simulink library "lib_fuel_cell"  (Simulink 4.00)
undefined symbols (not defined in the file or in its folder): air_cp, amb_tmp, cell_const_F, cell_const_g, cell_const_jo, cell_const_LHV_H2, cell_const_Mair, cell_const_MH, cell_const_MW, cell_const_R2, cell_const_Voc, ex_gas_cp, fan_cool, fc_acc_mass, fc_act, fc_air_comp_map, fc_air_comp_pwr, fc_base_mass, fc_blower_rec_H2, fc_blowera, fc_c2i_th_cond, fc_c_init_tmp, fc_cell_area, fc_cell_const_eta1, fc_cell_const_eta_DCDC, fc_cell_const_etablow, fc_cell_const_etagen, fc_cell_const_etapump, fc_cell_const_ex, fc_cell_const_kw, fc_cell_const_Nrad, fc_cell_const_U, fc_cell_dim_A, fc_cell_dim_tm, fc_cell_num, fc_cell_press_a, fc_cell_press_amb, fc_cell_press_an, fc_cell_press_blowa, fc_cell_press_blowr, fc_cell_press_c, fc_cell_press_hum, fc_cell_press_hyd, fc_cell_stack_dpipe, fc_cell_stack_dpipefc, fc_cell_stack_drad, fc_cell_stack_Lpipe, fc_cell_stack_Lpipefc, fc_cell_stack_Lrad, fc_cell_stack_N, fc_cell_stack_Pel, fc_cell_stoich_RHah, fc_cell_stoich_RHch, fc_cell_stoich_RHo, fc_cell_stoich_vH, fc_cell_stoich_vO, fc_cell_stoich_XON, fc_cell_temp_ah, fc_cell_temp_amb, fc_cell_temp_cell ... (+74)
libraries: fc_vt_lib x2, lib_fuel_cell x1
(part 3 of 5)

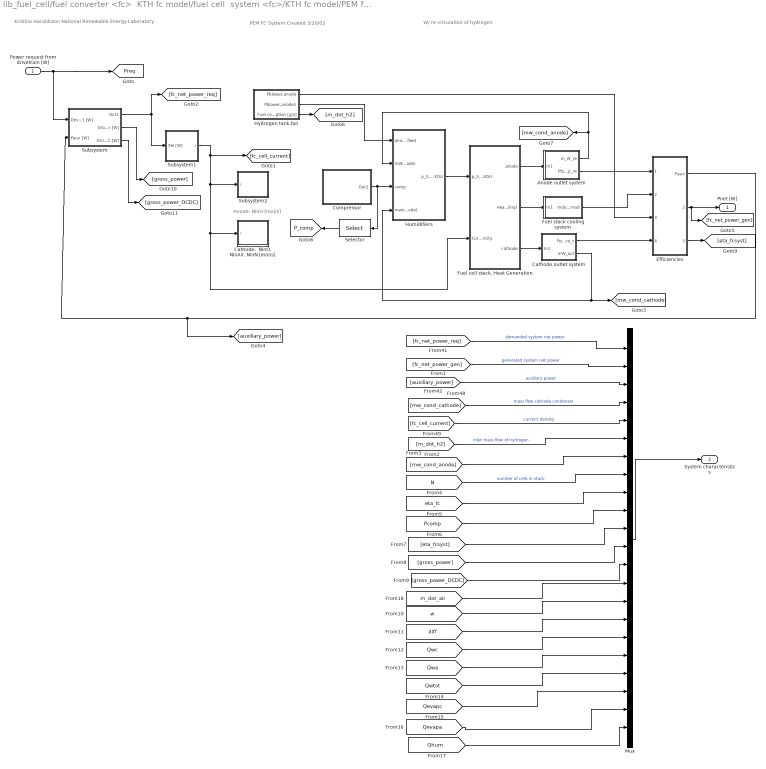
== system lib_fuel_cell/fuel converter <fc>  KTH fc model/fuel cell  system <fc>/KTH fc model/PEM fuel cell system ==
  note: Kristina Haraldsson
      | National Renewable Energy Laboratory
  note: PEM FC System
      | Created  3/20/02
  note: W/ re-circulation of hydrogen
  note: Anode: NinH [mol/s]
  "Power request from drivetrain [W] " : Inport  Port=1  LatchInput=off
  Anode outlet system : Subsystem
      settings: RTWFcnNameOpts=Auto  RTWFileNameOpts=Auto
  Cathode outlet system : Subsystem
      settings: RTWFcnNameOpts=Auto  RTWFileNameOpts=Auto
  "Cathode:  NinO, NinAir, NinN [mol/s]" : Subsystem
      settings: RTWFcnNameOpts=Auto  RTWFileNameOpts=Auto
  "Compressor " : Subsystem
      settings: RTWFcnNameOpts=Auto  RTWFileNameOpts=Auto
  Efficiencies : Subsystem
      settings: RTWFcnNameOpts=Auto  RTWFileNameOpts=Auto
  "Fuel cell stack, Heat Generation" : Subsystem
      settings: RTWFcnNameOpts=Auto  RTWFileNameOpts=Auto
  Fuel stack cooling system : Subsystem
      settings: RTWFcnNameOpts=Auto  RTWFileNameOpts=Auto
  Humidifiers : Subsystem
      settings: RTWFcnNameOpts=Auto  RTWFileNameOpts=Auto
  Hydrogen tank,fan : Subsystem
      settings: RTWFcnNameOpts=Auto  RTWFileNameOpts=Auto
  Mux : Mux  Inputs=22
  Selector : Selector  Orientation=left  InputType=Vector  ElementSrc=Internal  Elements=[4]  RowSrc=Internal  Rows=1  ColumnSrc=Internal  Columns=1  InputPortWidth=7
  Subsystem : Subsystem
      settings: RTWFcnNameOpts=Auto  RTWFileNameOpts=Auto
  Subsystem1 : Subsystem
      settings: RTWFcnNameOpts=Auto  RTWFileNameOpts=Auto
  Subsystem2 : Subsystem
      settings: RTWFcnNameOpts=Auto  RTWFileNameOpts=Auto
  Pnet [W] : Outport  Port=1
  System characteristics : Outport  Port=2
  tag scope: P_comp=global, Preq=global
  wires:
  Humidifiers/1("p_56 anode feed p_57 cathode feed Psat Psatah Psatch XWaI,  XWcI  XOcI ") -> "Fuel cell stack, Heat Generation"/1("p_56, NinH, p_57, NinAir, Psat,Psatah,PsatchXWaI, XWcI, XOcI")
  "Compressor "/1(Out2) -> Humidifiers/3(comp), Selector/1
  "Fuel cell stack, Heat Generation"/1(anode) -> Anode outlet system/1(In1)
  "Fuel cell stack, Heat Generation"/2(Heat_fc (fuel cell stack cooling)) -> Fuel stack cooling system/1(In1)
  Fuel stack cooling system/1(mdotW P_pump A Heat Qcool P_fanrad) -> Efficiencies/2(P_pump,cool P_fanrad)
  Anode outlet system/2(Pfan Ppump_re) -> Efficiencies/1("P_fan_,re, P_pump_re_a")
  Anode outlet system/1(m_W_re) -> Humidifiers/2(mW_out(anode)), [mw_cond_anode]
  "Fuel cell stack, Heat Generation"/3(cathode) -> Cathode outlet system/1(In1)
  Cathode outlet system/1(Ppump_re_c) -> Efficiencies/4(P_pump_re_c)
  Cathode outlet system/2(mW_out) -> Humidifiers/4(mwout(cathode)), [mw_cond_cathode]
  Hydrogen tank,fan/1(Pblower,anode) -> Efficiencies/3(P_fan,anode)
  Efficiencies/1(Paux) -> Subsystem/2(Paux [W]), [auxiliary_power]
  Subsystem/1(Out1) -> Subsystem1/1(Pel [W]), [fc_net_power_req]
  "Power request from drivetrain [W] "/1 -> Subsystem/1(Drivetrain Power Request [W]), [Preq]
  Subsystem1/1(i) -> Subsystem2/1(i), "Cathode:  NinO, NinAir, NinN [mol/s]"/1(i), "Fuel cell stack, Heat Generation"/2(Current density), [fc_cell_current]
  Hydrogen tank,fan/3(Fuel consumption [g/s]) -> [m_dot_h2]
  Hydrogen tank,fan/2(Pblower,anode1) -> Humidifiers/1(anode feed)
  [fc_net_power_req] -> Mux/1  "demanded system net power"
  [auxiliary_power] -> Mux/3  "auxiliary power"
  [mw_cond_cathode] -> Mux/4  "mass flow cathode condenser"
  [fc_cell_current] -> Mux/5  "current density"
  [fc_net_power_gen] -> Mux/2  "generated system net power"
  Mux/1 -> System characteristics/1
  [m_dot_h2] -> Mux/6  "inlet mass flow of hydrogen"
  [mw_cond_anode] -> Mux/7
  [N] -> Mux/8  "number of cells in stack"
  [eta_fc] -> Mux/9
  [Pcomp] -> Mux/10
  Selector/1 -> [P_comp]
  Subsystem/2(Gross power [W]) -> [gross_power]
  Efficiencies/2(Pnet [W]) -> Pnet [W]/1, [fc_net_power_gen]
  Efficiencies/3(eta_fcsyst) -> [eta_fcsyst]
  Subsystem/3(Gross power incl. DCDC [W]) -> [gross_power_DCDC]
  [eta_fcsyst] -> Mux/11
  [gross_power] -> Mux/12
  [gross_power_DCDC] -> Mux/13
  [Qhum] -> Mux/22
  [Qevapa] -> Mux/21
  [Qevapc] -> Mux/20
  [Qwtot] -> Mux/19
  [Qwa] -> Mux/18
  [Qwc] -> Mux/17
  [diff] -> Mux/16
  [w] -> Mux/15
  [m_dot_air] -> Mux/14

== system lib_fuel_cell/fuel converter <fc>  KTH fc model/fuel cell  system <fc>/KTH fc model/emissions info ==
  Block NOTES1 : Subsystem
      settings: RTWFcnNameOpts=Auto  RTWFileNameOpts=Auto
      mask Display: disp('Block\nNOTES')
  "CO, g/s1" : Ground
  Exhaust temp.=Cell temp. [C] : Constant  Value=fc_cell_temp_cell
  "HC, g/s2" : Ground
  Molecular weight H2 : Constant  Value=cell_const_MH
  Mux : Mux  Inputs=4
  Mux5 : Mux  Inputs=4
      settings: DisplayOption=none
  "NOx, g/s3" : Ground
  "O2, g/s" : Ground
  "PM, g/s4" : Ground
  Product : Product  Inputs=2  Multiplication=Element-wise(.*)  SaturateOnIntegerOverflow=on
  Sum : Sum  Inputs=|++  SaturateOnIntegerOverflow=on
  emission info CO HC NOx PM mass flow exhaust exhaust temperature O2 : Outport  Port=1  OutputWhenDisabled=reset  InitialOutput=eps
  wires:
  "O2, g/s"/1 -> Mux5/4
  Exhaust temp.=Cell temp. [C]/1 -> Mux5/3
  Mux5/1 -> emission info CO HC NOx PM mass flow exhaust exhaust temperature O2/1
  "CO, g/s1"/1 -> Mux/1
  Mux/1 -> Mux5/1
  "HC, g/s2"/1 -> Mux/2
  "NOx, g/s3"/1 -> Mux/3
  "PM, g/s4"/1 -> Mux/4
  Molecular weight H2/1 -> Product/1
  [Exhaust_a_hydrogen] -> Product/2
  Product/1 -> Sum/1
  [Exhaust_a_water] -> Sum/2
  Sum/1 -> Mux5/2

== system lib_fuel_cell/fuel converter <fc> GCTool linkage/fuel cell  system <fc>/GCTool fuel cell model/GCTool  Fuel Cell Model ==
  In1 : Inport  Port=1  LatchInput=off
  S-Function : S-Function  FunctionName=sfun_gctool_fuelcell  PortCounts=[]  SFunctionModules=''
  Out1 : Outport  Port=1  InitialOutput=0
  wires:
  S-Function/1 -> Out1/1
  In1/1 -> S-Function/1

== system lib_fuel_cell/fuel converter <fc> GCTool linkage/fuel use and EO emis Fuel Cell/fc temp/Block NOTES ==
  note: This block models the thermal behavior internal combustion engine (ICE).
      | Emphasis is on the coolant since this temperature is used to correct engine
      | fuel use.

== system lib_fuel_cell/fuel converter <fc> GCTool linkage/fuel use and EO emis Fuel Cell/fc temp/fc coolant ==
  Tcl : Inport  Port=1  LatchInput=off
  "Qfc_i " : Inport  Port=2  LatchInput=off
  Enable : EnablePort  StatesWhenEnabling=reset
  Constant : Constant  Value=fc_tstat
  Product1 : Product  Inputs=2  Multiplication=Element-wise(.*)  SaturateOnIntegerOverflow=on
  Qhtr : Fcn  Expr=fc_cl2h_eff*fc_h_air_flow*air_cp*(u - amb_tmp)
  Qi : Sum  Inputs=-+  SaturateOnIntegerOverflow=on
  Relational Operator : RelationalOperator  Operator=<=
  Qfc_rad : Outport  Port=1  OutputWhenDisabled=reset  InitialOutput=0
  Qfc_htr : Outport  Port=2  OutputWhenDisabled=reset  InitialOutput=0
  wires:
  Tcl/1 -> Qhtr/1, Relational Operator/2
  Relational Operator/1 -> Product1/1
  Constant/1 -> Relational Operator/1
  Product1/1 -> Qfc_rad/1
  "Qfc_i "/1 -> Qi/2
  Qhtr/1 -> Qi/1, Qfc_htr/1
  Qi/1 -> Product1/2

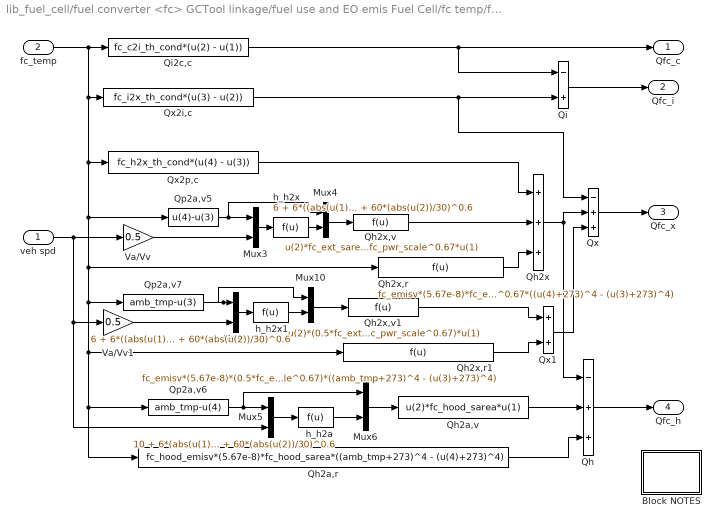
== system lib_fuel_cell/fuel converter <fc> GCTool linkage/fuel use and EO emis Fuel Cell/fc temp/fc mass heat flow ==
  veh spd : Inport  Port=1  LatchInput=off
  fc_temp : Inport  Port=2  LatchInput=off
  Block NOTES : Subsystem
      settings: RTWFcnNameOpts=Auto  RTWFileNameOpts=Auto
      mask Display: disp('Block\nNOTES')
  Mux{3..6,9..10} (6 alike) : Mux  Inputs=2
      settings: DisplayOption=none
  Qh : Sum  Inputs=-++  SaturateOnIntegerOverflow=on
  Qh2a,r : Fcn  Expr=fc_hood_emisv*(5.67e-8)*fc_hood_sarea*((amb_tmp+273)^4 - (u(4)+273)^4)
  Qh2a,v : Fcn  Expr=u(2)*fc_hood_sarea*u(1)
  Qh2x : Sum  Inputs=+++  SaturateOnIntegerOverflow=on
  Qh2x,r : Fcn  Expr=fc_emisv*(5.67e-8)*fc_ext_sarea*fc_pwr_scale^0.67*((u(4)+273)^4 - (u(3)+273)^4)
  Qh2x,r1 : Fcn  Expr=fc_emisv*(5.67e-8)*(0.5*fc_ext_sarea*fc_pwr_scale^0.67)*((amb_tmp+273)^4 - (u(3)+273)^4)
  Qh2x,v : Fcn  Expr=u(2)*fc_ext_sarea*fc_pwr_scale^0.67*u(1)
  Qh2x,v1 : Fcn  Expr=u(2)*(0.5*fc_ext_sarea*fc_pwr_scale^0.67)*u(1)
  Qi : Sum  Inputs=-+  SaturateOnIntegerOverflow=on
  Qi2c,c : Fcn  Expr=fc_c2i_th_cond*(u(2) - u(1))
  Qp2a,v5 : Fcn  Expr=u(4)-u(3)
  Qp2a,v6 : Fcn  Expr=amb_tmp-u(4)
  Qp2a,v7 : Fcn  Expr=amb_tmp-u(3)
  Qx : Sum  Inputs=-++  SaturateOnIntegerOverflow=on
  Qx1 : Sum  Inputs=++  SaturateOnIntegerOverflow=on
  Qx2i,c : Fcn  Expr=fc_i2x_th_cond*(u(3) - u(2))
  Qx2p,c : Fcn  Expr=fc_h2x_th_cond*(u(4) - u(3))
  Va/Vv : Gain  Gain=0.5  Multiplication=Element-wise(K.*u)  SaturateOnIntegerOverflow=on
  Va/Vv1 : Gain  Gain=0.5  Multiplication=Element-wise(K.*u)  SaturateOnIntegerOverflow=on
  h_h2a : Fcn  Expr=10 + 6*(abs(u(1))/1000)^0.3 + 60*(abs(u(2))/30)^0.6
  h_h2x : Fcn  Expr=6 + 6*((abs(u(1))/1000))^0.3 + 60*(abs(u(2))/30)^0.6
  h_h2x1 : Fcn  Expr=6 + 6*((abs(u(1))/1000))^0.3 + 60*(abs(u(2))/30)^0.6
  Qfc_c : Outport  Port=1
  Qfc_i : Outport  Port=2
  Qfc_x : Outport  Port=3
  Qfc_h : Outport  Port=4
  wires:
  Mux10/1 -> Qh2x,v1/1
  Mux9/1 -> h_h2x1/1
  Qp2a,v7/1 -> Mux9/1, Mux10/1
  h_h2x1/1 -> Mux10/2
  Va/Vv1/1 -> Mux9/2
  Mux4/1 -> Qh2x,v/1
  Mux3/1 -> h_h2x/1
  Qp2a,v5/1 -> Mux3/1, Mux4/1
  h_h2x/1 -> Mux4/2
  veh spd/1 -> Va/Vv/1, Mux5/2, Va/Vv1/1
  Va/Vv/1 -> Mux3/2
  Qi2c,c/1 -> Qfc_c/1, Qi/1
  fc_temp/1 -> Qx2p,c/1, Qh2x,r/1, Qp2a,v7/1, Qp2a,v6/1, Qh2a,r/1, Qh2x,r1/1, Qp2a,v5/1, Qx2i,c/1, Qi2c,c/1
  Qx2i,c/1 -> Qi/2, Qx/1
  Qi/1 -> Qfc_i/1
  Qx/1 -> Qfc_x/1
  Qh2x/1 -> Qx/2, Qh/1
  Qh/1 -> Qfc_h/1
  Mux6/1 -> Qh2a,v/1
  Mux5/1 -> h_h2a/1
  Qp2a,v6/1 -> Mux5/1, Mux6/1
  h_h2a/1 -> Mux6/2
  Qx1/1 -> Qx/3
  Qh2x,v/1 -> Qh2x/2
  Qx2p,c/1 -> Qh2x/1
  Qh2x,r1/1 -> Qx1/2
  Qh2x,v1/1 -> Qx1/1
  Qh2a,r/1 -> Qh/3
  Qh2a,v/1 -> Qh/2
  Qh2x,r/1 -> Qh2x/3

== system lib_fuel_cell/fuel converter <fc> GCTool linkage/fuel use and EO emis Fuel Cell/fc temp/old fc coolant  temp. (C) ==
  fc on? : Inport  Port=1  LatchInput=off
  veh spd : Inport  Port=2  LatchInput=off
  Block NOTES : Subsystem
      settings: RTWFcnNameOpts=Auto  RTWFileNameOpts=Auto
      mask Display: disp('Block\nNOTES')
  Mux : Mux  Inputs=4
      settings: DisplayOption=none
  TEC : Integrator  ExternalReset=none  InitialConditionSource=internal  InitialCondition=fc_i_init_tmp  LimitOutput=off  UpperSaturationLimit=inf  LowerSaturationLimit=-inf  ShowSaturationPort=off  ShowStatePort=off  AbsoluteTolerance=auto
  compute engine dT/dt : Fcn  Expr=1.1*u[1]*(-u[2]/218)*(95-u[4])+(1-u[1])*u[3]*(u[4]-amb_tmp)
  gamma (takes v as input) : Fcn  Expr=(-8.22e-5*u+8.09e-6*4-1.45e-4)*.45
  log(1-40/75) : Constant  Value=-0.7621
  fc coolant  temp (C) : Outport  Port=1  InitialOutput=0
  wires:
  compute engine dT/dt/1 -> TEC/1
  gamma (takes v as input)/1 -> Mux/3
  log(1-40/75)/1 -> Mux/2
  Mux/1 -> compute engine dT/dt/1
  fc on?/1 -> Mux/1
  veh spd/1 -> gamma (takes v as input)/1
  TEC/1 -> fc coolant  temp (C)/1, Mux/4

== system lib_fuel_cell/fuel converter <fc> VT model/Fuel Cell Power System Model (S. Gurski - Virgina Tech)/Fuel Cell System/Algebraic Constraint ==
  f(z) : Inport  Port=1  LatchInput=off
  Initial Guess : InitialCondition  Value=z0
  Sum : Sum  Inputs=|++  SaturateOnIntegerOverflow=on
  z : Outport  Port=1
  wires:
  Sum/1 -> Initial Guess/1
  Initial Guess/1 -> Sum/2, z/1
  f(z)/1 -> Sum/1

== system lib_fuel_cell/fuel converter <fc> VT model/Fuel Cell Power System Model (S. Gurski - Virgina Tech)/Fuel Cell System/Fuel Cell System ==
  " Current Density Request" : Inport  Port=1  LatchInput=off
  t_stack_coolant_in1 : Inport  Port=2  LatchInput=off
  fc_stack_temperature : Inport  Port=3  LatchInput=off
  water_balance_previous : Inport  Port=4  LatchInput=off
  elevation : Inport  Port=5  LatchInput=off
  vehicle speed (m/s) : Inport  Port=6  LatchInput=off
  Main Loop : fc_vt_lib/Main Loop
      settings: RTWFcnNameOpts=Auto  RTWFileNameOpts=Auto
  Net Power Gen : Outport  Port=1
  Stack Temperature : Outport  Port=2
  cell_voltage : Outport  Port=3
  t_stack_coolant_in : Outport  Port=4
  waterbalance : Outport  Port=5
  system_characteristics : Outport  Port=6
  wires:
  elevation/1 -> Main Loop/5
  Main Loop/6 -> system_characteristics/1
  water_balance_previous/1 -> Main Loop/4
  fc_stack_temperature/1 -> Main Loop/3
  t_stack_coolant_in1/1 -> Main Loop/2
  Main Loop/5 -> cell_voltage/1
  " Current Density Request"/1 -> Main Loop/1
  Main Loop/2 -> waterbalance/1
  Main Loop/3 -> Stack Temperature/1
  Main Loop/4 -> t_stack_coolant_in/1
  Main Loop/1 -> Net Power Gen/1
  vehicle speed (m/s)/1 -> Main Loop/6

== system lib_fuel_cell/fuel converter <fc> net model/fuel cell  system <fc>/pwr vs. eff  fuel cell model/enforce limits ==
  In1 : Inport  Port=1  LatchInput=off
  Saturation : Saturate  UpperLimit=max(fc_pwr_map)*fc_pwr_scale  LowerLimit=0  LinearizeAsGain=on
  Out1 : Outport  Port=1  InitialOutput=0
  wires:
  In1/1 -> Saturation/1
  Saturation/1 -> Out1/1

== system lib_fuel_cell/fuel converter <fc> net model/fuel use and EO emis Fuel Cell/HOT engine maps /Block NOTES ==
  note: This block determines the fully hot fuel use, engine-out emissions output rates, exhaust gas mass flow rate,
      | and engine-out exhaust gas temperature as a function of engine output torque and speed.
      | The engine maps (except for exhaust gas temperature) can be scaled using variables fc_spd_scale and
      |  fc_trq_scale; it is recommended that scaling values outside the range of 0.85 to 1.15 be used CAREFULLY.

== system lib_fuel_cell/fuel converter <fc> net model/fuel use and EO emis Fuel Cell/fc temp/Block NOTES ==
  note: This block models the thermal behavior internal combustion engine (ICE).
      | Emphasis is on the coolant since this temperature is used to correct engine
      | fuel use.

== system lib_fuel_cell/fuel converter <fc> net model/fuel use and EO emis Fuel Cell/fc temp/fc coolant ==
  Tcl : Inport  Port=1  LatchInput=off
  "Qfc_i " : Inport  Port=2  LatchInput=off
  Enable : EnablePort  StatesWhenEnabling=reset
  Constant : Constant  Value=fc_tstat
  Product1 : Product  Inputs=2  Multiplication=Element-wise(.*)  SaturateOnIntegerOverflow=on
  Qhtr : Fcn  Expr=fc_cl2h_eff*fc_h_air_flow*air_cp*(u - amb_tmp)
  Qi : Sum  Inputs=-+  SaturateOnIntegerOverflow=on
  Relational Operator : RelationalOperator  Operator=<=
  Qfc_rad : Outport  Port=1  OutputWhenDisabled=reset  InitialOutput=0
  Qfc_htr : Outport  Port=2  OutputWhenDisabled=reset  InitialOutput=0
  wires:
  Tcl/1 -> Qhtr/1, Relational Operator/2
  Relational Operator/1 -> Product1/1
  Constant/1 -> Relational Operator/1
  Product1/1 -> Qfc_rad/1
  "Qfc_i "/1 -> Qi/2
  Qhtr/1 -> Qi/1, Qfc_htr/1
  Qi/1 -> Product1/2

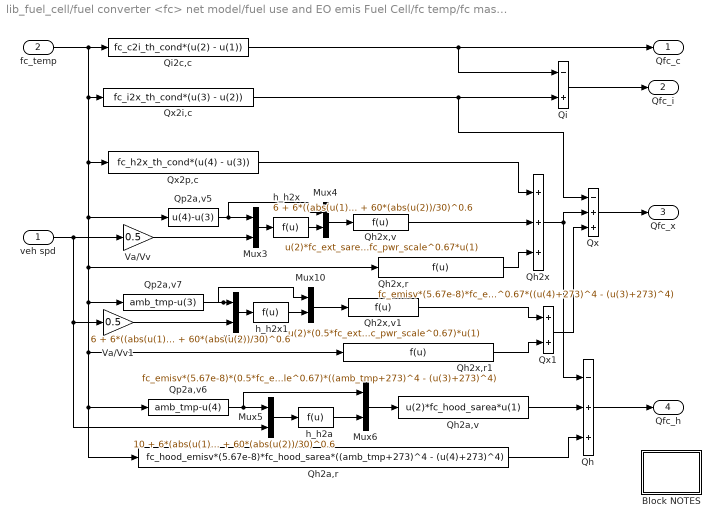
== system lib_fuel_cell/fuel converter <fc> net model/fuel use and EO emis Fuel Cell/fc temp/fc mass heat flow ==
  veh spd : Inport  Port=1  LatchInput=off
  fc_temp : Inport  Port=2  LatchInput=off
  Block NOTES : Subsystem
      settings: RTWFcnNameOpts=Auto  RTWFileNameOpts=Auto
      mask Display: disp('Block\nNOTES')
  Mux{3..6,9..10} (6 alike) : Mux  Inputs=2
      settings: DisplayOption=none
  Qh : Sum  Inputs=-++  SaturateOnIntegerOverflow=on
  Qh2a,r : Fcn  Expr=fc_hood_emisv*(5.67e-8)*fc_hood_sarea*((amb_tmp+273)^4 - (u(4)+273)^4)
  Qh2a,v : Fcn  Expr=u(2)*fc_hood_sarea*u(1)
  Qh2x : Sum  Inputs=+++  SaturateOnIntegerOverflow=on
  Qh2x,r : Fcn  Expr=fc_emisv*(5.67e-8)*fc_ext_sarea*fc_pwr_scale^0.67*((u(4)+273)^4 - (u(3)+273)^4)
  Qh2x,r1 : Fcn  Expr=fc_emisv*(5.67e-8)*(0.5*fc_ext_sarea*fc_pwr_scale^0.67)*((amb_tmp+273)^4 - (u(3)+273)^4)
  Qh2x,v : Fcn  Expr=u(2)*fc_ext_sarea*fc_pwr_scale^0.67*u(1)
  Qh2x,v1 : Fcn  Expr=u(2)*(0.5*fc_ext_sarea*fc_pwr_scale^0.67)*u(1)
  Qi : Sum  Inputs=-+  SaturateOnIntegerOverflow=on
  Qi2c,c : Fcn  Expr=fc_c2i_th_cond*(u(2) - u(1))
  Qp2a,v5 : Fcn  Expr=u(4)-u(3)
  Qp2a,v6 : Fcn  Expr=amb_tmp-u(4)
  Qp2a,v7 : Fcn  Expr=amb_tmp-u(3)
  Qx : Sum  Inputs=-++  SaturateOnIntegerOverflow=on
  Qx1 : Sum  Inputs=++  SaturateOnIntegerOverflow=on
  Qx2i,c : Fcn  Expr=fc_i2x_th_cond*(u(3) - u(2))
  Qx2p,c : Fcn  Expr=fc_h2x_th_cond*(u(4) - u(3))
  Va/Vv : Gain  Gain=0.5  Multiplication=Element-wise(K.*u)  SaturateOnIntegerOverflow=on
  Va/Vv1 : Gain  Gain=0.5  Multiplication=Element-wise(K.*u)  SaturateOnIntegerOverflow=on
  h_h2a : Fcn  Expr=10 + 6*(abs(u(1))/1000)^0.3 + 60*(abs(u(2))/30)^0.6
  h_h2x : Fcn  Expr=6 + 6*((abs(u(1))/1000))^0.3 + 60*(abs(u(2))/30)^0.6
  h_h2x1 : Fcn  Expr=6 + 6*((abs(u(1))/1000))^0.3 + 60*(abs(u(2))/30)^0.6
  Qfc_c : Outport  Port=1
  Qfc_i : Outport  Port=2
  Qfc_x : Outport  Port=3
  Qfc_h : Outport  Port=4
  wires:
  Mux10/1 -> Qh2x,v1/1
  Mux9/1 -> h_h2x1/1
  Qp2a,v7/1 -> Mux9/1, Mux10/1
  h_h2x1/1 -> Mux10/2
  Va/Vv1/1 -> Mux9/2
  Mux4/1 -> Qh2x,v/1
  Mux3/1 -> h_h2x/1
  Qp2a,v5/1 -> Mux3/1, Mux4/1
  h_h2x/1 -> Mux4/2
  veh spd/1 -> Va/Vv/1, Mux5/2, Va/Vv1/1
  Va/Vv/1 -> Mux3/2
  Qi2c,c/1 -> Qfc_c/1, Qi/1
  fc_temp/1 -> Qx2p,c/1, Qh2x,r/1, Qp2a,v7/1, Qp2a,v6/1, Qh2a,r/1, Qh2x,r1/1, Qp2a,v5/1, Qx2i,c/1, Qi2c,c/1
  Qx2i,c/1 -> Qi/2, Qx/1
  Qi/1 -> Qfc_i/1
  Qx/1 -> Qfc_x/1
  Qh2x/1 -> Qx/2, Qh/1
  Qh/1 -> Qfc_h/1
  Mux6/1 -> Qh2a,v/1
  Mux5/1 -> h_h2a/1
  Qp2a,v6/1 -> Mux5/1, Mux6/1
  h_h2a/1 -> Mux6/2
  Qx1/1 -> Qx/3
  Qh2x,v/1 -> Qh2x/2
  Qx2p,c/1 -> Qh2x/1
  Qh2x,r1/1 -> Qx1/2
  Qh2x,v1/1 -> Qx1/1
  Qh2a,r/1 -> Qh/3
  Qh2a,v/1 -> Qh/2
  Qh2x,r/1 -> Qh2x/3

== system lib_fuel_cell/fuel converter <fc> net model/fuel use and EO emis Fuel Cell/fc temp/old fc coolant  temp. (C) ==
  fc on? : Inport  Port=1  LatchInput=off
  veh spd : Inport  Port=2  LatchInput=off
  Block NOTES : Subsystem
      settings: RTWFcnNameOpts=Auto  RTWFileNameOpts=Auto
      mask Display: disp('Block\nNOTES')
  Mux : Mux  Inputs=4
      settings: DisplayOption=none
  TEC : Integrator  ExternalReset=none  InitialConditionSource=internal  InitialCondition=fc_i_init_tmp  LimitOutput=off  UpperSaturationLimit=inf  LowerSaturationLimit=-inf  ShowSaturationPort=off  ShowStatePort=off  AbsoluteTolerance=auto
  compute engine dT/dt : Fcn  Expr=1.1*u[1]*(-u[2]/218)*(95-u[4])+(1-u[1])*u[3]*(u[4]-amb_tmp)
  gamma (takes v as input) : Fcn  Expr=(-8.22e-5*u+8.09e-6*4-1.45e-4)*.45
  log(1-40/75) : Constant  Value=-0.7621
  fc coolant  temp (C) : Outport  Port=1  InitialOutput=0
  wires:
  compute engine dT/dt/1 -> TEC/1
  gamma (takes v as input)/1 -> Mux/3
  log(1-40/75)/1 -> Mux/2
  Mux/1 -> compute engine dT/dt/1
  fc on?/1 -> Mux/1
  veh spd/1 -> gamma (takes v as input)/1
  TEC/1 -> fc coolant  temp (C)/1, Mux/4

== system lib_fuel_cell/fuel converter <fc> net model/fuel use and EO emis Fuel Cell/fc temp correct/fc temp correct Constant Correction Factors (Equation Based) ==
  Coolant T (C) : Inport  Port=1  LatchInput=off
  HOT fuel use (g/s) : Inport  Port=2  LatchInput=off
  HOT emis (g/s) : Inport  Port=3  LatchInput=off
  Enable : EnablePort  StatesWhenEnabling=reset
  Block NOTES : Subsystem
      settings: RTWFcnNameOpts=Auto  RTWFileNameOpts=Auto
      mask Display: disp('Block\nNOTES')
  CO cold/hot : Fcn  Expr=2.13*pow(u,4.26)+1
  HC cold/hot : Fcn  Expr=8.05*pow(u,9.46)+1
  Mux : Mux  Inputs=4
      settings: DisplayOption=none
  NOx cold/hot : Fcn  Expr=0.51*pow(u,1.37)+1
  PM cold/hot : Fcn  Expr=5.14*pow(u,17.04)+1
  Product : Product  Inputs=2  Multiplication=Element-wise(.*)  SaturateOnIntegerOverflow=on
  Product1 : Product  Inputs=2  Multiplication=Element-wise(.*)  SaturateOnIntegerOverflow=on
  Saturation : Saturate  UpperLimit=1  LowerLimit=0  LinearizeAsGain=on
  fuel cold/hot : Fcn  Expr=0.1*pow(u,0.65)+1
  lambda : Fcn  Expr=(fc_tstat-u)/(fc_tstat-20)
  fuel use (g/s) : Outport  Port=1  OutputWhenDisabled=reset  InitialOutput=0
  EO emis (g/s) : Outport  Port=2  OutputWhenDisabled=reset  InitialOutput=0
  wires:
  HOT emis (g/s)/1 -> Product/2
  Coolant T (C)/1 -> lambda/1
  HOT fuel use (g/s)/1 -> Product1/1
  Product1/1 -> fuel use (g/s)/1
  CO cold/hot/1 -> Mux/2
  Product/1 -> EO emis (g/s)/1
  fuel cold/hot/1 -> Product1/2
  Mux/1 -> Product/1
  lambda/1 -> Saturation/1
  Saturation/1 -> PM cold/hot/1, NOx cold/hot/1, fuel cold/hot/1, HC cold/hot/1, CO cold/hot/1
  HC cold/hot/1 -> Mux/1
  NOx cold/hot/1 -> Mux/3
  PM cold/hot/1 -> Mux/4

== system lib_fuel_cell/fuel converter <fc> net model/fuel use and EO emis Fuel Cell/fc temp correct/fc temp correct Variable Correction Factors (Map Based) ==
  Coolant T (C) : Inport  Port=1  LatchInput=off
  HOT fuel use (g/s) : Inport  Port=2  LatchInput=off
  HOT emis (g/s) : Inport  Port=3  LatchInput=off
  P (W) : Inport  Port=4  LatchInput=off
  Enable : EnablePort  StatesWhenEnabling=reset
  (Thot-Temp) -------------------- (Thot-Tcold) : Fcn  Expr=(fc_tstat-u)/(fc_tstat-fc_cold_tmp)
  CO factor cold-to-hot : Lookup  InputValues=fc_pwr_map*fc_pwr_scale  OutputValues=fc_co_map_c2h
  HC factor cold-to-hot : Lookup  InputValues=fc_pwr_map*fc_pwr_scale  OutputValues=fc_hc_map_c2h
  Mux{1..5} (5 alike) : Mux  Inputs=2
      settings: DisplayOption=none
  Mux6 : Mux  Inputs=4
      settings: DisplayOption=none
  NOx factor cold-to-hot : Lookup  InputValues=fc_pwr_map*fc_pwr_scale  OutputValues=fc_nox_map_c2h
  PM factor cold-to-hot : Lookup  InputValues=fc_pwr_map*fc_pwr_scale  OutputValues=fc_pm_map_c2h
  Product : Product  Inputs=2  Multiplication=Element-wise(.*)  SaturateOnIntegerOverflow=on
  Product1 : Product  Inputs=2  Multiplication=Element-wise(.*)  SaturateOnIntegerOverflow=on
  Saturation : Saturate  UpperLimit=max(fc_pwr_map*fc_pwr_scale)  LowerLimit=0  LinearizeAsGain=on
  cold/hot =1+(factor-1) *Temp_ratio{,1..4} (5 alike) : Fcn  Expr=1+(u[2]-1)*u[1]
  fuel factor cold-to-hot : Lookup  InputValues=fc_pwr_map*fc_pwr_scale  OutputValues=fc_fuel_map_c2h
  limit to data limits : Saturate  UpperLimit=1  LowerLimit=0  LinearizeAsGain=on
  fuel use (g/s) : Outport  Port=1  OutputWhenDisabled=reset  InitialOutput=0
  EO emis (g/s) : Outport  Port=2  OutputWhenDisabled=reset  InitialOutput=0
  wires:
  cold/hot =1+(factor-1) *Temp_ratio4/1 -> Mux6/4
  cold/hot =1+(factor-1) *Temp_ratio3/1 -> Mux6/3
  cold/hot =1+(factor-1) *Temp_ratio2/1 -> Mux6/2
  cold/hot =1+(factor-1) *Temp_ratio1/1 -> Mux6/1
  cold/hot =1+(factor-1) *Temp_ratio/1 -> Product1/2
  limit to data limits/1 -> Mux1/1, Mux2/1, Mux3/1, Mux4/1, Mux5/1
  (Thot-Temp) -------------------- (Thot-Tcold)/1 -> limit to data limits/1
  Saturation/1 -> PM factor cold-to-hot/1, NOx factor cold-to-hot/1, CO factor cold-to-hot/1, HC factor cold-to-hot/1, fuel factor cold-to-hot/1
  P (W)/1 -> Saturation/1
  HOT fuel use (g/s)/1 -> Product1/1
  Coolant T (C)/1 -> (Thot-Temp) -------------------- (Thot-Tcold)/1
  fuel factor cold-to-hot/1 -> Mux1/2
  Mux1/1 -> cold/hot =1+(factor-1) *Temp_ratio/1
  HC factor cold-to-hot/1 -> Mux2/2
  CO factor cold-to-hot/1 -> Mux3/2
  NOx factor cold-to-hot/1 -> Mux4/2
  PM factor cold-to-hot/1 -> Mux5/2
  Mux2/1 -> cold/hot =1+(factor-1) *Temp_ratio1/1
  Mux3/1 -> cold/hot =1+(factor-1) *Temp_ratio2/1
  Mux4/1 -> cold/hot =1+(factor-1) *Temp_ratio3/1
  Mux5/1 -> cold/hot =1+(factor-1) *Temp_ratio4/1
  Product1/1 -> fuel use (g/s)/1
  Product/1 -> EO emis (g/s)/1
  HOT emis (g/s)/1 -> Product/2
  Mux6/1 -> Product/1

== system lib_fuel_cell/fuel converter <fc> polarization curve model/fuel cell  system <fc>/polarization curve fuel cell model/Auxilaries  (actual) ==
  In1 : Inport  Port=1  LatchInput=off
  Air Compressor : Subsystem
      settings: RTWFcnNameOpts=Auto  RTWFileNameOpts=Auto
  Coolant Pump : Subsystem
      settings: RTWFcnNameOpts=Auto  RTWFileNameOpts=Auto
  Fuel Pump : Subsystem
      settings: RTWFcnNameOpts=Auto  RTWFileNameOpts=Auto
  Mux : Mux  Inputs=4
  Water Pump : Subsystem
      settings: RTWFcnNameOpts=Auto  RTWFileNameOpts=Auto
  pwr sum1 : Sum  Inputs=++++  SaturateOnIntegerOverflow=on
  Out1 : Outport  Port=1  InitialOutput=0
  Out2 : Outport  Port=2  InitialOutput=0
  wires:
  Water Pump/1(water pump  pwr request (W)) -> pwr sum1/3, Mux/3
  Coolant Pump/1(coolant pump  pwr request (W)) -> pwr sum1/4, Mux/4
  Air Compressor/1(air compressor  pwr request (W)) -> pwr sum1/2, Mux/2
  Fuel Pump/1(fuel pump  pwr request (W)) -> pwr sum1/1, Mux/1
  pwr sum1/1 -> Out1/1
  In1/1 -> Air Compressor/1(Fuel req'd (g/s)), Fuel Pump/1(Fuel req'd (g/s)), Water Pump/1(Fuel req'd (g/s))
  Mux/1 -> Out2/1

== system lib_fuel_cell/fuel converter <fc> polarization curve model/fuel cell  system <fc>/polarization curve fuel cell model/Auxilaries  (estimated) ==
  prev fuel  req (g/s) : Inport  Port=1  LatchInput=off
  Air Compressor : Subsystem
      settings: RTWFcnNameOpts=Auto  RTWFileNameOpts=Auto
  Coolant Pump : Subsystem
      settings: RTWFcnNameOpts=Auto  RTWFileNameOpts=Auto
  Fuel Pump : Subsystem
      settings: RTWFcnNameOpts=Auto  RTWFileNameOpts=Auto
  Water Pump : Subsystem
      settings: RTWFcnNameOpts=Auto  RTWFileNameOpts=Auto
  pwr sum : Sum  Inputs=++++  SaturateOnIntegerOverflow=on
  Aux pwr req'd (W) : Outport  Port=1  InitialOutput=0
  wires:
  pwr sum/1 -> Aux pwr req'd (W)/1
  Coolant Pump/1(coolant pump  pwr request (W)) -> pwr sum/4
  Water Pump/1(water pump  pwr request (W)) -> pwr sum/3
  Air Compressor/1(air compressor  pwr request (W)) -> pwr sum/2
  Fuel Pump/1(fuel pump  pwr request (W)) -> pwr sum/1
  prev fuel  req (g/s)/1 -> Air Compressor/1(Fuel req'd (g/s)), Fuel Pump/1(Fuel req'd (g/s)), Water Pump/1(Fuel req'd (g/s))

== system lib_fuel_cell/fuel converter <fc> polarization curve model/fuel cell  system <fc>/polarization curve fuel cell model/Fuel Cell Stack ==
  Pack pwr req : Inport  Port=1  LatchInput=off
  *cell_area : Gain  Gain=fc_cell_area  Multiplication=Element-wise(K.*u)  SaturateOnIntegerOverflow=on
  *fc_cell_num *fc_stack_num : Gain  Gain=fc_cell_num*fc_stack_num  Multiplication=Element-wise(K.*u)  SaturateOnIntegerOverflow=on
  *fc_cell_num *fc_stack_num *fc_string_num : Gain  Gain=fc_stack_num*fc_string_num*fc_cell_num  Multiplication=Element-wise(K.*u)  SaturateOnIntegerOverflow=on
  *string_num : Gain  Gain=fc_string_num  Multiplication=Element-wise(K.*u)  SaturateOnIntegerOverflow=on
  Block NOTES : Subsystem
      settings: RTWFcnNameOpts=Auto  RTWFileNameOpts=Auto
      mask Display: disp('Block\nNOTES')
  Mux : Mux  Inputs=7
  P --------------------- (strings*stacks*fc_cell_num*cell_area) : Gain  Gain=1/fc_string_num/fc_stack_num/fc_cell_num/fc_cell_area  Multiplication=Element-wise(K.*u)  SaturateOnIntegerOverflow=on
  Product2 : Product  Inputs=2  Multiplication=Element-wise(.*)  SaturateOnIntegerOverflow=on
  Product3 : Product  Inputs=*/  Multiplication=Element-wise(.*)  SaturateOnIntegerOverflow=on
  Sum2 : Sum  Inputs=-+  SaturateOnIntegerOverflow=on
  Sum3 : Sum  Inputs=-+  SaturateOnIntegerOverflow=on
  cell voltage : Lookup  InputValues=fc_I_map*fc_pwr_scale  OutputValues=fc_V_map
  current density : Lookup  InputValues=fc_I_map.*fc_V_map*fc_pwr_scale  OutputValues=fc_I_map*fc_pwr_scale
  emissions info : Subsystem
      settings: RTWFcnNameOpts=Auto  RTWFileNameOpts=Auto
  enforce limits : Subsystem
      settings: RTWFcnNameOpts=Auto  RTWFileNameOpts=Auto
  fuel flow (g/s) : Lookup  InputValues=fc_I_map*fc_pwr_scale  OutputValues=fc_fuel_map*fc_pwr_scale/fc_eff_scale
  utilization  factor : Lookup  InputValues=fc_I_map*fc_pwr_scale  OutputValues=fc_fuel_utilization_map
  gross pwr out a (W) : Outport  Port=1  InitialOutput=0
  fuel used (g/s) : Outport  Port=2  InitialOutput=0
  emis info : Outport  Port=3  InitialOutput=0
  diagnostics : Outport  Port=4  InitialOutput=0
  wires:
  emissions info/1(emis  info) -> emis info/1
  current density/1 -> enforce limits/1(In1)
  enforce limits/1(Out1) -> emissions info/1(current density (amps/m^2)), *cell_area/1, Mux/2, cell voltage/1, utilization  factor/1, fuel flow (g/s)/1
  P --------------------- (strings*stacks*fc_cell_num*cell_area)/1 -> current density/1
  fuel flow (g/s)/1 -> *fc_cell_num *fc_stack_num *fc_string_num/1
  Sum3/1 -> fuel used (g/s)/1
  *fc_cell_num *fc_stack_num/1 -> Product2/1, Mux/6
  cell voltage/1 -> *fc_cell_num *fc_stack_num/1, Mux/5
  *string_num/1 -> Product2/2, Mux/4
  Sum2/1 -> Sum3/1, Mux/7
  *fc_cell_num *fc_stack_num *fc_string_num/1 -> Sum3/2, Sum2/1, Product3/1
  Product3/1 -> Sum2/2
  utilization  factor/1 -> Product3/2
  *cell_area/1 -> *string_num/1, Mux/3
  Pack pwr req/1 -> P --------------------- (strings*stacks*fc_cell_num*cell_area)/1, Mux/1
  Mux/1 -> diagnostics/1
  Product2/1 -> gross pwr out a (W)/1

== system lib_fuel_cell/fuel converter <fc> polarization curve model/fuel use and EO emis Fuel Cell/fc temp/Block NOTES ==
  note: This block models the thermal behavior internal combustion engine (ICE).
      | Emphasis is on the coolant since this temperature is used to correct engine
      | fuel use.

== system lib_fuel_cell/fuel converter <fc> polarization curve model/fuel use and EO emis Fuel Cell/fc temp/fc coolant ==
  Tcl : Inport  Port=1  LatchInput=off
  "Qfc_i " : Inport  Port=2  LatchInput=off
  Enable : EnablePort  StatesWhenEnabling=reset
  Constant : Constant  Value=fc_tstat
  Product1 : Product  Inputs=2  Multiplication=Element-wise(.*)  SaturateOnIntegerOverflow=on
  Qhtr : Fcn  Expr=fc_cl2h_eff*fc_h_air_flow*air_cp*(u - amb_tmp)
  Qi : Sum  Inputs=-+  SaturateOnIntegerOverflow=on
  Relational Operator : RelationalOperator  Operator=<=
  Qfc_rad : Outport  Port=1  OutputWhenDisabled=reset  InitialOutput=0
  Qfc_htr : Outport  Port=2  OutputWhenDisabled=reset  InitialOutput=0
  wires:
  Tcl/1 -> Qhtr/1, Relational Operator/2
  Relational Operator/1 -> Product1/1
  Constant/1 -> Relational Operator/1
  Product1/1 -> Qfc_rad/1
  "Qfc_i "/1 -> Qi/2
  Qhtr/1 -> Qi/1, Qfc_htr/1
  Qi/1 -> Product1/2

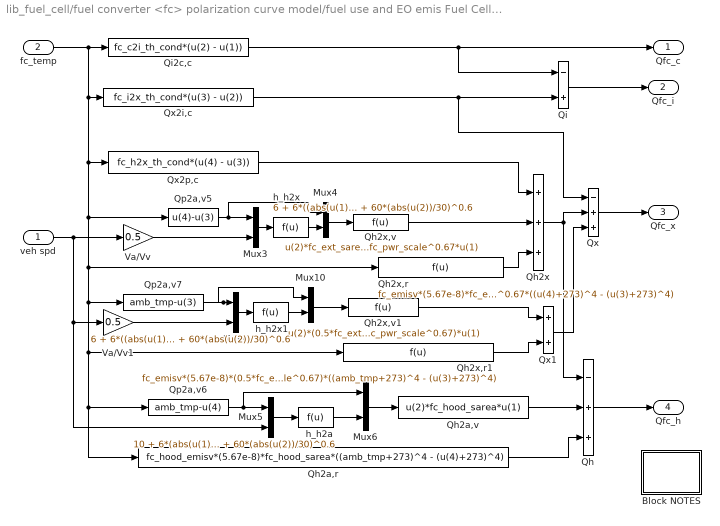
== system lib_fuel_cell/fuel converter <fc> polarization curve model/fuel use and EO emis Fuel Cell/fc temp/fc mass heat flow ==
  veh spd : Inport  Port=1  LatchInput=off
  fc_temp : Inport  Port=2  LatchInput=off
  Block NOTES : Subsystem
      settings: RTWFcnNameOpts=Auto  RTWFileNameOpts=Auto
      mask Display: disp('Block\nNOTES')
  Mux{3..6,9..10} (6 alike) : Mux  Inputs=2
      settings: DisplayOption=none
  Qh : Sum  Inputs=-++  SaturateOnIntegerOverflow=on
  Qh2a,r : Fcn  Expr=fc_hood_emisv*(5.67e-8)*fc_hood_sarea*((amb_tmp+273)^4 - (u(4)+273)^4)
  Qh2a,v : Fcn  Expr=u(2)*fc_hood_sarea*u(1)
  Qh2x : Sum  Inputs=+++  SaturateOnIntegerOverflow=on
  Qh2x,r : Fcn  Expr=fc_emisv*(5.67e-8)*fc_ext_sarea*fc_pwr_scale^0.67*((u(4)+273)^4 - (u(3)+273)^4)
  Qh2x,r1 : Fcn  Expr=fc_emisv*(5.67e-8)*(0.5*fc_ext_sarea*fc_pwr_scale^0.67)*((amb_tmp+273)^4 - (u(3)+273)^4)
  Qh2x,v : Fcn  Expr=u(2)*fc_ext_sarea*fc_pwr_scale^0.67*u(1)
  Qh2x,v1 : Fcn  Expr=u(2)*(0.5*fc_ext_sarea*fc_pwr_scale^0.67)*u(1)
  Qi : Sum  Inputs=-+  SaturateOnIntegerOverflow=on
  Qi2c,c : Fcn  Expr=fc_c2i_th_cond*(u(2) - u(1))
  Qp2a,v5 : Fcn  Expr=u(4)-u(3)
  Qp2a,v6 : Fcn  Expr=amb_tmp-u(4)
  Qp2a,v7 : Fcn  Expr=amb_tmp-u(3)
  Qx : Sum  Inputs=-++  SaturateOnIntegerOverflow=on
  Qx1 : Sum  Inputs=++  SaturateOnIntegerOverflow=on
  Qx2i,c : Fcn  Expr=fc_i2x_th_cond*(u(3) - u(2))
  Qx2p,c : Fcn  Expr=fc_h2x_th_cond*(u(4) - u(3))
  Va/Vv : Gain  Gain=0.5  Multiplication=Element-wise(K.*u)  SaturateOnIntegerOverflow=on
  Va/Vv1 : Gain  Gain=0.5  Multiplication=Element-wise(K.*u)  SaturateOnIntegerOverflow=on
  h_h2a : Fcn  Expr=10 + 6*(abs(u(1))/1000)^0.3 + 60*(abs(u(2))/30)^0.6
  h_h2x : Fcn  Expr=6 + 6*((abs(u(1))/1000))^0.3 + 60*(abs(u(2))/30)^0.6
  h_h2x1 : Fcn  Expr=6 + 6*((abs(u(1))/1000))^0.3 + 60*(abs(u(2))/30)^0.6
  Qfc_c : Outport  Port=1
  Qfc_i : Outport  Port=2
  Qfc_x : Outport  Port=3
  Qfc_h : Outport  Port=4
  wires:
  Mux10/1 -> Qh2x,v1/1
  Mux9/1 -> h_h2x1/1
  Qp2a,v7/1 -> Mux9/1, Mux10/1
  h_h2x1/1 -> Mux10/2
  Va/Vv1/1 -> Mux9/2
  Mux4/1 -> Qh2x,v/1
  Mux3/1 -> h_h2x/1
  Qp2a,v5/1 -> Mux3/1, Mux4/1
  h_h2x/1 -> Mux4/2
  veh spd/1 -> Va/Vv/1, Mux5/2, Va/Vv1/1
  Va/Vv/1 -> Mux3/2
  Qi2c,c/1 -> Qfc_c/1, Qi/1
  fc_temp/1 -> Qx2p,c/1, Qh2x,r/1, Qp2a,v7/1, Qp2a,v6/1, Qh2a,r/1, Qh2x,r1/1, Qp2a,v5/1, Qx2i,c/1, Qi2c,c/1
  Qx2i,c/1 -> Qi/2, Qx/1
  Qi/1 -> Qfc_i/1
  Qx/1 -> Qfc_x/1
  Qh2x/1 -> Qx/2, Qh/1
  Qh/1 -> Qfc_h/1
  Mux6/1 -> Qh2a,v/1
  Mux5/1 -> h_h2a/1
  Qp2a,v6/1 -> Mux5/1, Mux6/1
  h_h2a/1 -> Mux6/2
  Qx1/1 -> Qx/3
  Qh2x,v/1 -> Qh2x/2
  Qx2p,c/1 -> Qh2x/1
  Qh2x,r1/1 -> Qx1/2
  Qh2x,v1/1 -> Qx1/1
  Qh2a,r/1 -> Qh/3
  Qh2a,v/1 -> Qh/2
  Qh2x,r/1 -> Qh2x/3

== system lib_fuel_cell/fuel converter <fc> polarization curve model/fuel use and EO emis Fuel Cell/fc temp/old fc coolant  temp. (C) ==
  fc on? : Inport  Port=1  LatchInput=off
  veh spd : Inport  Port=2  LatchInput=off
  Block NOTES : Subsystem
      settings: RTWFcnNameOpts=Auto  RTWFileNameOpts=Auto
      mask Display: disp('Block\nNOTES')
  Mux : Mux  Inputs=4
      settings: DisplayOption=none
  TEC : Integrator  ExternalReset=none  InitialConditionSource=internal  InitialCondition=fc_i_init_tmp  LimitOutput=off  UpperSaturationLimit=inf  LowerSaturationLimit=-inf  ShowSaturationPort=off  ShowStatePort=off  AbsoluteTolerance=auto
  compute engine dT/dt : Fcn  Expr=1.1*u[1]*(-u[2]/218)*(95-u[4])+(1-u[1])*u[3]*(u[4]-amb_tmp)
  gamma (takes v as input) : Fcn  Expr=(-8.22e-5*u+8.09e-6*4-1.45e-4)*.45
  log(1-40/75) : Constant  Value=-0.7621
  fc coolant  temp (C) : Outport  Port=1  InitialOutput=0
  wires:
  compute engine dT/dt/1 -> TEC/1
  gamma (takes v as input)/1 -> Mux/3
  log(1-40/75)/1 -> Mux/2
  Mux/1 -> compute engine dT/dt/1
  fc on?/1 -> Mux/1
  veh spd/1 -> gamma (takes v as input)/1
  TEC/1 -> fc coolant  temp (C)/1, Mux/4

== system lib_fuel_cell/fuel converter <fc> polarization curve model/fuel use and EO emis Fuel Cell/fc temp correct/fc temp correct Constant Correction Factors (Equation Based) ==
  Coolant T (C) : Inport  Port=1  LatchInput=off
  HOT fuel use (g/s) : Inport  Port=2  LatchInput=off
  HOT emis (g/s) : Inport  Port=3  LatchInput=off
  Enable : EnablePort  StatesWhenEnabling=reset
  Block NOTES : Subsystem
      settings: RTWFcnNameOpts=Auto  RTWFileNameOpts=Auto
      mask Display: disp('Block\nNOTES')
  CO cold/hot : Fcn  Expr=2.13*pow(u,4.26)+1
  HC cold/hot : Fcn  Expr=8.05*pow(u,9.46)+1
  Mux : Mux  Inputs=4
      settings: DisplayOption=none
  NOx cold/hot : Fcn  Expr=0.51*pow(u,1.37)+1
  PM cold/hot : Fcn  Expr=5.14*pow(u,17.04)+1
  Product : Product  Inputs=2  Multiplication=Element-wise(.*)  SaturateOnIntegerOverflow=on
  Product1 : Product  Inputs=2  Multiplication=Element-wise(.*)  SaturateOnIntegerOverflow=on
  Saturation : Saturate  UpperLimit=1  LowerLimit=0  LinearizeAsGain=on
  fuel cold/hot : Fcn  Expr=0.1*pow(u,0.65)+1
  lambda : Fcn  Expr=(fc_tstat-u)/(fc_tstat-20)
  fuel use (g/s) : Outport  Port=1  OutputWhenDisabled=reset  InitialOutput=0
  EO emis (g/s) : Outport  Port=2  OutputWhenDisabled=reset  InitialOutput=0
  wires:
  HOT emis (g/s)/1 -> Product/2
  Coolant T (C)/1 -> lambda/1
  HOT fuel use (g/s)/1 -> Product1/1
  Product1/1 -> fuel use (g/s)/1
  CO cold/hot/1 -> Mux/2
  Product/1 -> EO emis (g/s)/1
  fuel cold/hot/1 -> Product1/2
  Mux/1 -> Product/1
  lambda/1 -> Saturation/1
  Saturation/1 -> PM cold/hot/1, NOx cold/hot/1, fuel cold/hot/1, HC cold/hot/1, CO cold/hot/1
  HC cold/hot/1 -> Mux/1
  NOx cold/hot/1 -> Mux/3
  PM cold/hot/1 -> Mux/4

== system lib_fuel_cell/fuel converter <fc> polarization curve model/fuel use and EO emis Fuel Cell/fc temp correct/fc temp correct Variable Correction Factors (Map Based) ==
  Coolant T (C) : Inport  Port=1  LatchInput=off
  HOT fuel use (g/s) : Inport  Port=2  LatchInput=off
  HOT emis (g/s) : Inport  Port=3  LatchInput=off
  P (W) : Inport  Port=4  LatchInput=off
  Enable : EnablePort  StatesWhenEnabling=reset
  (Thot-Temp) -------------------- (Thot-Tcold) : Fcn  Expr=(fc_tstat-u)/(fc_tstat-fc_cold_tmp)
  CO factor cold-to-hot : Lookup  InputValues=fc_pwr_map*fc_pwr_scale  OutputValues=fc_co_map_c2h
  HC factor cold-to-hot : Lookup  InputValues=fc_pwr_map*fc_pwr_scale  OutputValues=fc_hc_map_c2h
  Mux{1..5} (5 alike) : Mux  Inputs=2
      settings: DisplayOption=none
  Mux6 : Mux  Inputs=4
      settings: DisplayOption=none
  NOx factor cold-to-hot : Lookup  InputValues=fc_pwr_map*fc_pwr_scale  OutputValues=fc_nox_map_c2h
  PM factor cold-to-hot : Lookup  InputValues=fc_pwr_map*fc_pwr_scale  OutputValues=fc_pm_map_c2h
  Product : Product  Inputs=2  Multiplication=Element-wise(.*)  SaturateOnIntegerOverflow=on
  Product1 : Product  Inputs=2  Multiplication=Element-wise(.*)  SaturateOnIntegerOverflow=on
  Saturation : Saturate  UpperLimit=max(fc_pwr_map*fc_pwr_scale)  LowerLimit=0  LinearizeAsGain=on
  cold/hot =1+(factor-1) *Temp_ratio{,1..4} (5 alike) : Fcn  Expr=1+(u[2]-1)*u[1]
  fuel factor cold-to-hot : Lookup  InputValues=fc_pwr_map*fc_pwr_scale  OutputValues=fc_fuel_map_c2h
  limit to data limits : Saturate  UpperLimit=1  LowerLimit=0  LinearizeAsGain=on
  fuel use (g/s) : Outport  Port=1  OutputWhenDisabled=reset  InitialOutput=0
  EO emis (g/s) : Outport  Port=2  OutputWhenDisabled=reset  InitialOutput=0
  wires:
  cold/hot =1+(factor-1) *Temp_ratio4/1 -> Mux6/4
  cold/hot =1+(factor-1) *Temp_ratio3/1 -> Mux6/3
  cold/hot =1+(factor-1) *Temp_ratio2/1 -> Mux6/2
  cold/hot =1+(factor-1) *Temp_ratio1/1 -> Mux6/1
  cold/hot =1+(factor-1) *Temp_ratio/1 -> Product1/2
  limit to data limits/1 -> Mux1/1, Mux2/1, Mux3/1, Mux4/1, Mux5/1
  (Thot-Temp) -------------------- (Thot-Tcold)/1 -> limit to data limits/1
  Saturation/1 -> PM factor cold-to-hot/1, NOx factor cold-to-hot/1, CO factor cold-to-hot/1, HC factor cold-to-hot/1, fuel factor cold-to-hot/1
  P (W)/1 -> Saturation/1
  HOT fuel use (g/s)/1 -> Product1/1
  Coolant T (C)/1 -> (Thot-Temp) -------------------- (Thot-Tcold)/1
  fuel factor cold-to-hot/1 -> Mux1/2
  Mux1/1 -> cold/hot =1+(factor-1) *Temp_ratio/1
  HC factor cold-to-hot/1 -> Mux2/2
  CO factor cold-to-hot/1 -> Mux3/2
  NOx factor cold-to-hot/1 -> Mux4/2
  PM factor cold-to-hot/1 -> Mux5/2
  Mux2/1 -> cold/hot =1+(factor-1) *Temp_ratio1/1
  Mux3/1 -> cold/hot =1+(factor-1) *Temp_ratio2/1
  Mux4/1 -> cold/hot =1+(factor-1) *Temp_ratio3/1
  Mux5/1 -> cold/hot =1+(factor-1) *Temp_ratio4/1
  Product1/1 -> fuel use (g/s)/1
  Product/1 -> EO emis (g/s)/1
  HOT emis (g/s)/1 -> Product/2
  Mux6/1 -> Product/1

== system lib_fuel_cell/fuel converter <fc>  KTH fc model/fuel cell  system <fc>/KTH fc model/PEM fuel cell system/Anode outlet system ==
  note: Anode outlet system
  In1 : Inport  Port=1  LatchInput=off
  Anode condenser : Subsystem
      settings: RTWFcnNameOpts=Auto  RTWFileNameOpts=Auto
  Mux : Mux  Inputs=2
  Mux1 : Mux  Inputs=2
  "Re-circulation: Blower_rec, pump" : Subsystem
      settings: RTWFcnNameOpts=Auto  RTWFileNameOpts=Auto
  Vent/Purge : Subsystem
      settings: RTWFcnNameOpts=Auto  RTWFileNameOpts=Auto
  m_W_re : Outport  Port=1
  Pfan Ppump_re : Outport  Port=2
  tag scope: NoutH=global
  wires:
  In1/1 -> Anode condenser/1(In1)
  Anode condenser/1(Out1) -> Vent/Purge/1(In1)
  Vent/Purge/1(Out1) -> "Re-circulation: Blower_rec, pump"/1(In1)
  "Re-circulation: Blower_rec, pump"/3(p_70) -> Mux/2
  "Re-circulation: Blower_rec, pump"/4(Pfan) -> Mux1/1
  "Re-circulation: Blower_rec, pump"/5(Ppump_re) -> Mux1/2
  Mux1/1 -> Pfan Ppump_re/1
  "Re-circulation: Blower_rec, pump"/1(m_W_re) -> m_W_re/1
  "Re-circulation: Blower_rec, pump"/2(NoutH_re) -> Mux/1
  Mux/1 -> [NoutH]

== system lib_fuel_cell/fuel converter <fc>  KTH fc model/fuel cell  system <fc>/KTH fc model/PEM fuel cell system/Cathode outlet system ==
  note: Cathode outlet system
  In1 : Inport  Port=1  LatchInput=off
  Cathode condenser : Subsystem
      settings: RTWFcnNameOpts=Auto  RTWFileNameOpts=Auto
  Pump (cathode) : Subsystem
      settings: RTWFcnNameOpts=Auto  RTWFileNameOpts=Auto
  Ppump_re_c : Outport  Port=1
  mW_out : Outport  Port=2
  wires:
  In1/1 -> Cathode condenser/1(In1)
  Pump (cathode)/1(Ppump_re_c) -> Ppump_re_c/1
  Cathode condenser/1(mw_out1) -> Pump (cathode)/1(In1)
  Pump (cathode)/2(mW_out) -> mW_out/1

== system lib_fuel_cell/fuel converter <fc>  KTH fc model/fuel cell  system <fc>/KTH fc model/PEM fuel cell system/Cathode:  NinO, NinAir, NinN [mol/s] ==
  note: Total cathode molar flow
  i : Inport  Port=1  LatchInput=off
  Constant : Constant  Value=fc_cell_stoich_vO
  Constant1 : Constant  Value=fc_cell_dim_A
  Constant2 : Constant  Value=fc_cell_stack_N
  Constant3 : Constant  Value=cell_const_F
  Constant4 : Constant  Value=4
  Constant5 : Constant  Value=fc_cell_stoich_XON
  Constant6 : Constant  Value=fc_cell_stoich_XON
  Constant7 : Constant  Value=1
  Constant8 : Constant  Value=cell_const_Mair
  Product : Product  Inputs=4  Multiplication=Element-wise(.*)  SaturateOnIntegerOverflow=on
  Product1 : Product  Inputs=*/  Multiplication=Element-wise(.*)  SaturateOnIntegerOverflow=on
  Product2 : Product  Inputs=2  Multiplication=Element-wise(.*)  SaturateOnIntegerOverflow=on
  Product3 : Product  Inputs=*/  Multiplication=Element-wise(.*)  SaturateOnIntegerOverflow=on
  Product4 : Product  Inputs=2  Multiplication=Element-wise(.*)  SaturateOnIntegerOverflow=on
  Product5 : Product  Inputs=2  Multiplication=Element-wise(.*)  SaturateOnIntegerOverflow=on
  Sum : Sum  Inputs=|+-  SaturateOnIntegerOverflow=on
  tag scope: NinAir=global, NinN=global, NinO=global, m_dot_air=global
  wires:
  Constant1/1 -> Product/3
  Constant/1 -> Product/2
  i/1 -> Product/1
  Constant2/1 -> Product/4
  Product/1 -> Product1/1
  Constant4/1 -> Product2/2
  Product2/1 -> Product1/2
  Product1/1 -> Product3/1, [NinO]
  Constant5/1 -> Product3/2
  Product3/1 -> Product4/1, Product5/1, [NinAir]
  Constant7/1 -> Sum/1
  Constant6/1 -> Sum/2
  Sum/1 -> Product4/2
  Product4/1 -> [NinN]
  Constant3/1 -> Product2/1
  Constant8/1 -> Product5/2
  Product5/1 -> [m_dot_air]

== system lib_fuel_cell/fuel converter <fc>  KTH fc model/fuel cell  system <fc>/KTH fc model/PEM fuel cell system/Compressor  ==
  note: Compressor
  Cathode pressure : Constant  Value=fc_cell_press_c
  "Initial value, 0.1 mole/s" : Memory  X0=0.1  InheritSampleTime=off
      settings: RTWStateStorageClass=Auto
  M_air [g/mol] : Constant  Value=cell_const_Mair
  Mass flow [g/s]  discharge pressure [bar(a)] CompOA1050 (Opcon) : Lookup  InputValues=[Qm_1050]  OutputValues=[p2_1050]
  Mass flow [g/s] Pcomp [W] CompOA1050 (Opcon) : Lookup  InputValues=[Qm_1050]  OutputValues=[Pcomp_1050]
  Mass flow [g/s] discharge temperature [C] CompOA1050 (Opcon)1 : Lookup  InputValues=[Qm_1050]  OutputValues=[T2_1050]
  Mux : Mux  Inputs=5
  Product : Product  Inputs=2  Multiplication=Element-wise(.*)  SaturateOnIntegerOverflow=on
  fc_compressor.m : MATLABFcn  MATLABFcn=fc_compressor(u,fc_cell_press_amb,fc_cell_temp_amb,fc_cell_const_eta1,fc_cell_const_etagen,fc_cell_stoich_RHo,fc_cell_press_hum,fc_cell_temp_evap,fc_cell_temp_cell,fc_cell_stack_Pel)  OutputDimensions=7  OutputSignalType=auto  Output1D=on
  Out2 : Outport  Port=1
  wires:
  M_air [g/mol]/1 -> Product/2
  Mux/1 -> fc_compressor.m/1
  fc_compressor.m/1 -> Out2/1
  Mass flow [g/s]  discharge pressure [bar(a)] CompOA1050 (Opcon)/1 -> Mux/2
  Mass flow [g/s] Pcomp [W] CompOA1050 (Opcon)/1 -> Mux/3
  [NinAir] -> "Initial value, 0.1 mole/s"/1
  "Initial value, 0.1 mole/s"/1 -> Mux/1, Product/1
  Product/1 -> Mass flow [g/s]  discharge pressure [bar(a)] CompOA1050 (Opcon)/1, Mass flow [g/s] Pcomp [W] CompOA1050 (Opcon)/1, Mass flow [g/s] discharge temperature [C] CompOA1050 (Opcon)1/1
  Mass flow [g/s] discharge temperature [C] CompOA1050 (Opcon)1/1 -> Mux/4
  Cathode pressure/1 -> Mux/5

== system lib_fuel_cell/fuel converter <fc>  KTH fc model/fuel cell  system <fc>/KTH fc model/PEM fuel cell system/Efficiencies ==
  note: Efficiencies
  "P_fan_,re, P_pump_re_a" : Inport  Port=1  LatchInput=off
  P_pump,cool P_fanrad : Inport  Port=2  LatchInput=off
  P_fan,anode : Inport  Port=3  LatchInput=off
  P_pump_re_c : Inport  Port=4  LatchInput=off
  Constant : Constant  Value=cell_const_LHV_H2
  Demux : Demux  Outputs=2  BusSelectionMode=off
  Demux1 : Demux  Outputs=2  BusSelectionMode=off
  Product : Product  Inputs=*/  Multiplication=Element-wise(.*)  SaturateOnIntegerOverflow=on
  Product1 : Product  Inputs=2  Multiplication=Element-wise(.*)  SaturateOnIntegerOverflow=on
  Selector1 : Selector  InputType=Vector  ElementSrc=Internal  Elements=[2 6]  RowSrc=Internal  Rows=1  ColumnSrc=Internal  Columns=1  InputPortWidth=6
  Sum{,1..6} (7 alike) : Sum  Inputs=|++  SaturateOnIntegerOverflow=on
  Sum7 : Sum  Inputs=|-+  SaturateOnIntegerOverflow=on
  Paux : Outport  Port=1
  Pnet [W] : Outport  Port=2
  eta_fcsyst : Outport  Port=3
  tag scope: Pcomp=global
  wires:
  P_pump,cool P_fanrad/1 -> Selector1/1
  [P_comp] -> Sum/1, [Pcomp]
  "P_fan_,re, P_pump_re_a"/1 -> Demux/1
  P_pump_re_c/1 -> Sum6/2
  P_fan,anode/1 -> Sum5/2
  Demux/1 -> Sum3/2
  Demux/2 -> Sum4/2
  [P_fancool] -> Sum/2
  Sum/1 -> Sum1/1
  Selector1/1 -> Demux1/1
  Demux1/1 -> Sum1/2
  Sum1/1 -> Sum2/1
  Demux1/2 -> Sum2/2
  Sum2/1 -> Sum3/1
  Sum3/1 -> Sum4/1
  Sum4/1 -> Sum5/1
  Sum5/1 -> Sum6/1
  Sum6/1 -> Sum7/1, Paux/1
  Sum7/1 -> Product/1, Pnet [W]/1
  [Preq] -> Sum7/2
  Constant/1 -> Product1/2
  [NinH] -> Product1/1
  Product1/1 -> Product/2
  Product/1 -> eta_fcsyst/1

== system lib_fuel_cell/fuel converter <fc>  KTH fc model/fuel cell  system <fc>/KTH fc model/PEM fuel cell system/Fuel cell stack, Heat Generation ==
  note: FCSystem_H2
      | /Fuel cell stack, Heat generation
  note: NinWa NinHa NoutWag NoutHa
      | NinWc NinO NinN NoutWcg NWlgen
      | NoutWcl NoutO NoutN Nout_condc Nout_conda
  "p_56, NinH, p_57, NinAir, Psat,Psatah,PsatchXWaI, XWcI, XOcI" : Inport  Port=1  LatchInput=off
  Current density : Inport  Port=2  LatchInput=off
  Constant1 : Constant  Value=cell_const_F
  Constant3 : Constant  Value=2
  Heat : Subsystem
      settings: RTWFcnNameOpts=Auto  RTWFileNameOpts=Auto
  J Water produced at cathode : Product  Inputs=/*  Multiplication=Element-wise(.*)  SaturateOnIntegerOverflow=on
  Mux1 : Mux  Inputs=5
  Product2 : Product  Inputs=2  Multiplication=Element-wise(.*)  SaturateOnIntegerOverflow=on
  fc_eqs : MATLABFcn  MATLABFcn=fc_eqs(u,fc_cell_dim_A,fc_cell_press_a,fc_cell_press_c,fc_cell_press_amb,fc_cell_stoich_RHo,cell_const_F,fc_cell_temp_cell,fc_cell_temp_ah,fc_cell_temp_ch,fc_cell_temp_amb,fc_cell_membrane_Mm,fc_cell_membrane_pdry,fc_cell_dim_tm,fc_cell_stoich_vO,fc_cell_stoich_vH,fc_cell_const_zw,fc_cell_stack_Pel,fc_cell_stack_N)  OutputDimensions=20  OutputSignalType=auto  Output1D=on
  flows : Selector  InputType=Vector  ElementSrc=Internal  Elements=[3 4 5 6 7 8 10 11 12 13 14 19 20]  RowSrc=Internal  Rows=1  ColumnSrc=Internal  Columns=1  InputPortWidth=20
  flows p_60 NoutWcg NoutWlgen NoutWcl NoutO NoutN Nout_condc : Selector  InputType=Vector  ElementSrc=Internal  Elements=[1 10 11 12 13 14 19]  RowSrc=Internal  Rows=1  ColumnSrc=Internal  Columns=1  InputPortWidth=20
  "p_61,NoutWag, NoutHa,NWAout,NoutWal" : Selector  InputType=Vector  ElementSrc=Internal  Elements=[2 5 6 16 17]  RowSrc=Internal  Rows=1  ColumnSrc=Internal  Columns=1  InputPortWidth=20
  anode : Outport  Port=1
  Heat_fc (fuel cell stack cooling) : Outport  Port=2
  cathode : Outport  Port=3
  tag scope: eta_fc=global
  wires:
  "p_56, NinH, p_57, NinAir, Psat,Psatah,PsatchXWaI, XWcI, XOcI"/1 -> Mux1/1
  "p_61,NoutWag, NoutHa,NWAout,NoutWal"/1 -> anode/1
  Mux1/1 -> fc_eqs/1
  fc_eqs/1 -> "p_61,NoutWag, NoutHa,NWAout,NoutWal"/1, flows/1, flows p_60 NoutWcg NoutWlgen NoutWcl NoutO NoutN Nout_condc/1
  flows/1 -> Heat/1(In1 NinWa NinHa NoutWag NoutHa NinWc NinO NinN NoutWcg NoutWcl NoutO NoutN Nout_condc Nout_conda)
  Heat/1(Heat_fc) -> Heat_fc (fuel cell stack cooling)/1
  [NinO] -> Mux1/2
  [NinN] -> Mux1/3
  [lambda] -> Mux1/4
  Current density/1 -> Heat/2(Current density [A/cm2]), J Water produced at cathode/2
  Heat/2(eta_fc) -> [eta_fc]
  flows p_60 NoutWcg NoutWlgen NoutWcl NoutO NoutN Nout_condc/1 -> cathode/1
  Constant1/1 -> Product2/1
  Constant3/1 -> Product2/2
  Product2/1 -> J Water produced at cathode/1
  J Water produced at cathode/1 -> Mux1/5
